simulink model "MultirotorPathFollowing"  (R2025b)
settings: Solver=FixedStepAuto  StartTime=0.0  StopTime=5  FixedStep=1e-4  RelTol=1e-3
undefined symbols (not defined in the file): convertStringsToChars, initialState
libraries: slpidlib x3, uavutilslib x1, uavalgslib x1
settings Model: SimulationMode=accelerator  Creator=Admin  LastModifiedBy=Admin

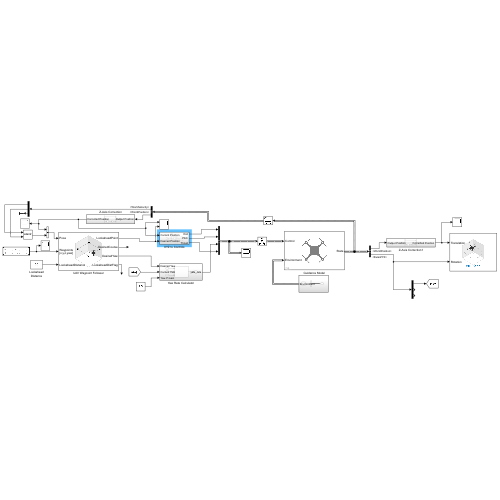
[thumbnail: Simulink's stored preview of the top-level diagram]
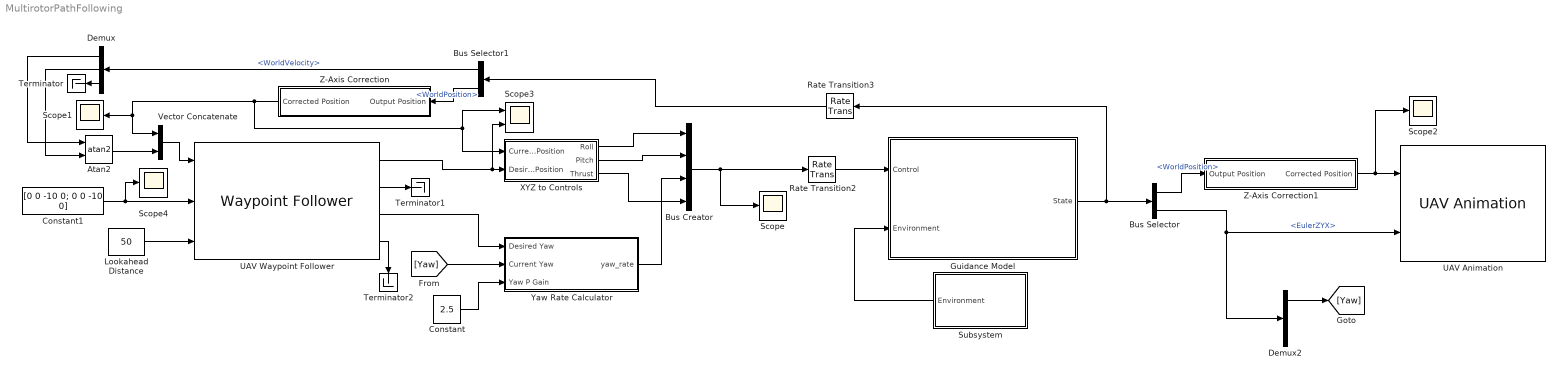
== system MultirotorPathFollowing ==
  Atan2 : Trigonometry  Operator=atan2
  Bus Creator : BusCreator  Inputs=4  OutDataTypeStr=Bus: MultirotorGuidanceControlBus  NonVirtualBus=on
      settings: InheritFromInputs=off
  Bus Selector : BusSelector  OutputSignals=WorldPosition,EulerZYX
  Bus Selector1 : BusSelector  OutputSignals=WorldVelocity,WorldPosition
  Constant : Constant  Value=2.5
  Constant1 : Constant  Value=[0 0 -10 0; 0 0 -10 0]  OutDataTypeStr=Inherit: Inherit via back propagation  SampleTime=-1
  Demux : Demux  Outputs=3
  Demux2 : Demux  Outputs=3
  Guidance Model : Subsystem  AncestorBlock=uavalgslib/Guidance Model  mask(Guidance Model){ModelType=MultirotorGuidance, NumInstances=1, SpecifiedDataType=double, SimulateUsing=Interpreted execution, InitialWorldPositionMultirotor=[0; 0; 10], InitialWorldVelocityMultirotor=[0; 0; 0], InitialEulerZYXMultirotor=[0; 0; 0], InitialBodyAngularRateRPYMultirotor=[0; 0; 0], InitialThrustMultirotor=0, InitialNorthFixedWing=0, InitialEastFixedWing=0, InitialHeightFixedWing=0, InitialAirSpeedFixedWing=0, InitialHeadingAngleFixedWing=0, InitialFlightPathAngleFixedWing=0, InitialRollAngleFixedWing=0, InitialRollAngleRateFixedWing=0, PDRollMultirotor=[3402.97,116.67], PDPitchMultirotor=[3402.97, 116.67], PYawRateMultirotor=1950, PThrustMultirotor=3900, MassMultirotor=2, PHeightFixedWing=3.9, PHeadingAngleFixedWing=3.9, PFlightPathAngleFixedWing=39, PDRollFixedWing=[3402.97, 116.67], PAirSpeedFixedWing=1, FlightPathAngleLimitsFixedWing=[-pi/2, pi/2], StateBusName='MultirotorGuidanceStateBus', ControlBusName='MultirotorGuidanceControlBus', EnvironmentBusName='MultirotorGuidanceEnvironmentBus', DataType=double}
      mask prompts: ModelType "uav:robotsluav:guidancemodelblock:ModelType"; NumInstances "Number of Instances:"; SpecifiedDataType "uav:robotsluav:guidancemodelblock:DataType"; SimulateUsing "SystemBlock:MATLABSystem:SimulateUsing"; InitialWorldPositionMultirotor "uav:robotsluav:guidancemodelblock:WorldPosition"; InitialWorldVelocityMultirotor "uav:robotsluav:guidancemodelblock:WorldVelocity"; InitialEulerZYXMultirotor "uav:robotsluav:guidancemodelblock:EulerZYX"; InitialBodyAngularRateRPYMultirotor "uav:robotsluav:guidancemodelblock:BodyAngularRateRPY"; InitialThrustMultirotor "uav:robotsluav:guidancemodelblock:Thrust"; InitialNorthFixedWing "uav:robotsluav:guidancemodelblock:NorthPosition"; InitialEastFixedWing "uav:robotsluav:guidancemodelblock:EastPosition"; InitialHeightFixedWing "uav:robotsluav:guidancemodelblock:Height"; InitialAirSpeedFixedWing "uav:robotsluav:guidancemodelblock:AirSpeed"; InitialHeadingAngleFixedWing "uav:robotsluav:guidancemodelblock:HeadingAngle"; InitialFlightPathAngleFixedWing "uav:robotsluav:guidancemodelblock:FlightPathAngle"; InitialRollAngleFixedWing "uav:robotsluav:guidancemodelblock:RollAngle"; InitialRollAngleRateFixedWing "uav:robotsluav:guidancemodelblock:RollAngleRate"; PDRollMultirotor "uav:robotsluav:guidancemodelblock:PDRoll"; PDPitchMultirotor "uav:robotsluav:guidancemodelblock:PDPitch"; PYawRateMultirotor "uav:robotsluav:guidancemodelblock:PYawRate"; PThrustMultirotor "uav:robotsluav:guidancemodelblock:PThrust"; MassMultirotor "uav:robotsluav:guidancemodelblock:Mass"; PHeightFixedWing "uav:robotsluav:guidancemodelblock:PHeight"; PHeadingAngleFixedWing "uav:robotsluav:guidancemodelblock:PHeadingAngle"; PFlightPathAngleFixedWing "uav:robotsluav:guidancemodelblock:PFlightPathAngle"; PDRollFixedWing "uav:robotsluav:guidancemodelblock:PDRollAngle"; PAirSpeedFixedWing "uav:robotsluav:guidancemodelblock:PAirSpeed"; FlightPathAngleLimitsFixedWing "uav:robotsluav:guidancemodelblock:MinMaxFlightPathAngle"; StateBusName "uav:robotsluav:guidancemodelblock:StateBusName"; ControlBusName "uav:robotsluav:guidancemodelblock:ControlBusName"; EnvironmentBusName "uav:robotsluav:guidancemodelblock:EnvironmentBusName"; DataType "uav:robotsluav:guidancemodelblock:ResolvedDataType"
      mask help: uav:robotsluav:guidancemodelblock:Description
      mask init:
      | ModelName = gcb;
      | 
      | % Validate bus names
      | uav.sluav.internal.guidancemodel.mask.validateBusNames(gcb);
      | 
      | [stateDimension, initialState, UAVType, UAVDataType, UAVConfig] = ...
      |     uav.sluav.internal.guidancemodel.mask.initialize(ModelName, ModelType, gcb, NumInstances);
      mask Help: eval('helpview(''uav'', ''uavGuidanceModelBlock'')');
      mask TypeOptions ModelType: uav:robotsluav:guidancemodelblock:ModelTypeMultirotor | uav:robotsluav:guidancemodelblock:ModelTypeFixedWing
      mask Callback ModelType:
      | % Change mask dialog
      | uav.sluav.internal.guidancemodel.mask.modelTypeCallback(gcb);
      | 
      | % Create buses for the UAV block
      | uav.sluav.internal.guidancemodel.mask.createUAVBuses(gcb);
      mask Callback SpecifiedDataType:
      | if ~strcmp(get_param(gcb, 'SpecifiedDataType'), '<data type expression>')
      |     % Resolve input type
      |     uav.sluav.internal.guidancemodel.mask.dataTypeCallback(gcb);
      | 
      |     % Create buses for the UAV block
      |     uav.sluav.internal.guidancemodel.mask.createUAVBuses(gcb);
      | end
      mask TypeOptions SimulateUsing: ComputeDerivative/SimulateUsing | StateVector2Struct/SimulateUsing
      mask Callback StateBusName:
      | % Validate bus names
      | uav.sluav.internal.guidancemodel.mask.validateBusNames(gcb);
      | 
      | % Create buses for the UAV block
      | uav.sluav.internal.guidancemodel.mask.createUAVBuses(gcb);
      mask Callback ControlBusName:
      | % Validate bus names
      | uav.sluav.internal.guidancemodel.mask.validateBusNames(gcb);
      | 
      | % Create buses for the UAV block
      | uav.sluav.internal.guidancemodel.mask.createUAVBuses(gcb);
      mask Callback EnvironmentBusName:
      | % Validate bus names
      | uav.sluav.internal.guidancemodel.mask.validateBusNames(gcb);
      | 
      | % Create buses for the UAV block
      | uav.sluav.internal.guidancemodel.mask.createUAVBuses(gcb);
      mask DialogControl ModelType Prompt: Model Type:
      mask DialogControl SpecifiedDataType Prompt: Data Type:
      mask DialogControl SimulateUsing Prompt: Simulate using:
      mask DialogControl SimulateUsing Tooltip: SystemBlock:MATLABSystem:SimulateUsingDescription
      mask DialogControl InitialStateTab Prompt: uav:robotsluav:guidancemodelblock:InitialState
      mask DialogControl InitialWorldPositionMultirotor Prompt: World Position
      mask DialogControl InitialWorldVelocityMultirotor Prompt: World Velocity
      mask DialogControl InitialEulerZYXMultirotor Prompt: Euler Angles (ZYX)
      mask DialogControl InitialBodyAngularRateRPYMultirotor Prompt: Body Angular Rate
      mask DialogControl InitialThrustMultirotor Prompt: Thrust
      mask DialogControl InitialNorthFixedWing Prompt: North Position
      mask DialogControl InitialEastFixedWing Prompt: East Position
      mask DialogControl InitialHeightFixedWing Prompt: Height
      mask DialogControl InitialAirSpeedFixedWing Prompt: Air Speed
      mask DialogControl InitialHeadingAngleFixedWing Prompt: Heading Angle
      mask DialogControl InitialFlightPathAngleFixedWing Prompt: Flight Path Angle
      mask DialogControl InitialRollAngleFixedWing Prompt: Roll Angle
      mask DialogControl InitialRollAngleRateFixedWing Prompt: Roll Angular Velocity
      mask DialogControl ConfigurationTab Prompt: uav:robotsluav:guidancemodelblock:Configuration
      mask DialogControl PDRollMultirotor Prompt: PD Roll
      mask DialogControl PDPitchMultirotor Prompt: PD Pitch
      mask DialogControl PYawRateMultirotor Prompt: P YawRate
      mask DialogControl PThrustMultirotor Prompt: P Thrust
      mask DialogControl MassMultirotor Prompt: Mass
      mask DialogControl PHeightFixedWing Prompt: P Height
      mask DialogControl PHeadingAngleFixedWing Prompt: P Heading Angle
      mask DialogControl PFlightPathAngleFixedWing Prompt: P Flight Path Angle
      mask DialogControl PDRollFixedWing Prompt: PD Roll Angle
      mask DialogControl PAirSpeedFixedWing Prompt: P Air Speed
      mask DialogControl FlightPathAngleLimitsFixedWing Prompt: Min/Max Flight Path Angle
      mask DialogControl BusNameTab Prompt: uav:robotsluav:guidancemodelblock:InputOutputBusNames
      mask DialogControl StateBusName Prompt: State Bus Name
      mask DialogControl ControlBusName Prompt: Control Bus Name
      mask DialogControl EnvironmentBusName Prompt: Environment Bus Name
      mask DialogControl DataType Prompt: Resolved Data Type
      mask Display:
      | port_label('input', 1, 'Control')
      | port_label('input', 2, 'Environment')
      | port_label('output', 1, 'State')
  Lookahead Distance : Constant  Value=50
  Rate Transition2 : RateTransition  OutPortSampleTime=0.1
  Rate Transition3 : RateTransition  OutPortSampleTime=0.1
  Scope{,1..2,4} (4 alike) : Scope
      Scope settings: ActiveDisplayYMinimum=-1  ActiveDisplayYMaximum=1
      Scope1 settings: ActiveDisplayYMinimum=-1  ActiveDisplayYMaximum=1
      Scope2 settings: ActiveDisplayYMinimum=-1  ActiveDisplayYMaximum=1  DataLoggingVariableName=ScopeData2
      Scope4 settings: ActiveDisplayYMinimum=-2.4999999999999996  ActiveDisplayYMaximum=22.5  DataLoggingVariableName=ScopeData4
  Scope3 : Scope  NumInputPorts=2
      settings: ActiveDisplayYMinimum=-481.410610510493  ActiveDisplayYMaximum=53.490067834499207  DataLoggingVariableName=ScopeData3
  Subsystem : Subsystem
  Terminator : Terminator
  Terminator1 : Terminator
  Terminator2 : Terminator
  UAV Animation : uavutilslib/UAV Animation  NumUAV=1  DynamicUAVConfig=off  UAVType=Multirotor  UAVSize=1  UAVColor=[1 0 0]  UAVTrajectoryAlpha=1  InertialZDirection=Down  RotationFormat=Euler ZYX  DrawMarkers=off  SampleTime=-1
  UAV Waypoint Follower : uavalgslib/Waypoint Follower  UAVType=multirotor  StartFrom=first  TransitionRadiusSource=internal  TransitionRadius=10  MinLookaheadDistance=0.1  HoverAtLastWaypoint=off  YawInput=on  ShowCrossTrackErrorOutput=off  ShowStatusOutput=off  SimulateUsing=Code generation
  Vector Concatenate : Concatenate
  XYZ to Controls : Subsystem
  Yaw Rate Calculator : Subsystem
  Z-Axis Correction : Subsystem
  Z-Axis Correction1 : Subsystem
  wires:
  Subsystem/1(Environment) -> Guidance Model/2(Environment)
  Rate Transition2/1 -> Guidance Model/1(Control)
  Guidance Model/1(State) -> Rate Transition3/1, Bus Selector/1
  Bus Selector/2 -> Demux2/1, UAV Animation/2  "<EulerZYX>"
  Lookahead Distance/1 -> UAV Waypoint Follower/3
  Rate Transition3/1 -> Bus Selector1/1
  Vector Concatenate/1 -> UAV Waypoint Follower/1
  Bus Selector1/1 -> Demux/1  "<WorldVelocity>"
  Demux/1 -> Atan2/1
  Demux/2 -> Atan2/2
  Atan2/1 -> Vector Concatenate/2
  Demux/3 -> Terminator/1
  UAV Waypoint Follower/4 -> Terminator2/1
  Bus Creator/1 -> Scope/1, Rate Transition2/1
  UAV Waypoint Follower/3 -> Yaw Rate Calculator/1(Desired Yaw)
  Demux2/1 -> [Yaw]
  [Yaw] -> Yaw Rate Calculator/2("Current Yaw ")
  Constant/1 -> Yaw Rate Calculator/3(Yaw P Gain)
  Yaw Rate Calculator/1(yaw_rate) -> Bus Creator/3
  UAV Waypoint Follower/1 -> Scope3/2, XYZ to Controls/2(Desired Position)
  XYZ to Controls/1(Roll) -> Bus Creator/1
  XYZ to Controls/2(Pitch) -> Bus Creator/2
  XYZ to Controls/3(Thrust) -> Bus Creator/4
  Constant1/1 -> Scope4/1, UAV Waypoint Follower/2
  Bus Selector1/2 -> Z-Axis Correction/1(Output Position)  "<WorldPosition>"
  Z-Axis Correction/1(Corrected Position) -> Scope3/1, XYZ to Controls/1(Current Position), Scope1/1, Vector Concatenate/1
  Z-Axis Correction1/1(Corrected Position) -> Scope2/1, UAV Animation/1
  Bus Selector/1 -> Z-Axis Correction1/1(Output Position)  "<WorldPosition>"
  UAV Waypoint Follower/2 -> Terminator1/1

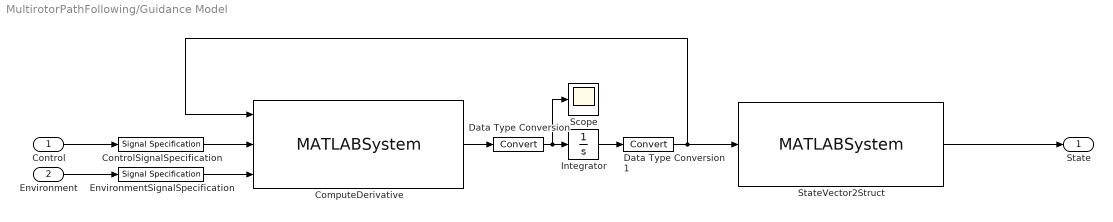
== system MultirotorPathFollowing/Guidance Model ==
  Control : Inport
  Environment : Inport  Port=2
  ComputeDerivative : MATLABSystem  System=robotics.core.internal.system.navigation.Model  ModelName=ModelName  ModelType=UAVType  ModelConfiguration=UAVConfig  DataType=UAVDataType  UseExternalConfiguration=false  NumInstances=NumInstances  SimulateUsing=Interpreted execution
      mask Type: robotics.core.internal.system.navigation.Model
  ControlSignalSpecification : SignalSpecification  OutDataTypeStr=Bus: MultirotorGuidanceControlBus  BusOutputAsStruct=on
  Data Type Conversion : DataTypeConversion  SaturateOnIntegerOverflow=off  RndMeth=Floor
  Data Type Conversion1 : DataTypeConversion  SaturateOnIntegerOverflow=off  RndMeth=Floor
  EnvironmentSignalSpecification : SignalSpecification  OutDataTypeStr=Bus: MultirotorGuidanceEnvironmentBus  BusOutputAsStruct=on
  Integrator : Integrator  InitialCondition=double(initialState)
  Scope : Scope
      settings: ActiveDisplayYMinimum=-20321.068651257519  ActiveDisplayYMaximum=4289.4123209348782  DataLoggingVariableName=ScopeData6
  StateVector2Struct : MATLABSystem  System=robotics.core.internal.system.navigation.StateVector2Struct  OutputBusName=convertStringsToChars(StateBusName)  ModelType=UAVType  DataType=UAVDataType  NumInstances=NumInstances  SimulateUsing=Interpreted execution
      mask Type: robotics.core.internal.system.navigation.StateVector2Struct
  State : Outport  VectorParamsAs1DForOutWhenUnconnected=off  BusOutputAsStruct=on
  wires:
  EnvironmentSignalSpecification/1 -> ComputeDerivative/3
  ControlSignalSpecification/1 -> ComputeDerivative/2
  Data Type Conversion1/1 -> ComputeDerivative/1, StateVector2Struct/1
  Data Type Conversion/1 -> Scope/1, Integrator/1
  Environment/1 -> EnvironmentSignalSpecification/1
  Control/1 -> ControlSignalSpecification/1
  Integrator/1 -> Data Type Conversion1/1
  ComputeDerivative/1 -> Data Type Conversion/1
  StateVector2Struct/1 -> State/1

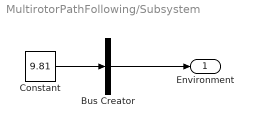
== system MultirotorPathFollowing/Subsystem ==
  Bus Creator : BusCreator  Inputs=1  OutDataTypeStr=Bus: MultirotorGuidanceEnvironmentBus  NonVirtualBus=on
      settings: InheritFromInputs=off
  Constant : Constant  Value=9.81
  Environment : Outport
  wires:
  Bus Creator/1 -> Environment/1
  Constant/1 -> Bus Creator/1

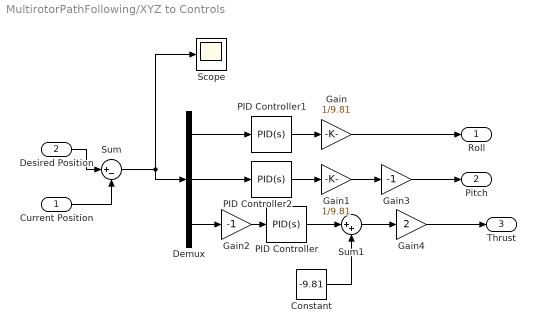
== system MultirotorPathFollowing/XYZ to Controls ==
  Current Position : Inport
  Desired Position : Inport  Port=2
  Constant : Constant  Value=-9.81
  Demux : Demux  Outputs=3
  Gain : Gain  Gain=1/9.81
  Gain1 : Gain  Gain=1/9.81
  Gain2 : Gain  Gain=-1
  Gain3 : Gain  Gain=-1
  Gain4 : Gain  Gain=2
  PID Controller : slpidlib/PID Controller  Controller=PID  Form=Parallel  TimeDomain=Continuous-time  UseExternalTs=off  SampleTime=-1  IntegratorMethod=Forward Euler  FilterMethod=Forward Euler  ControllerParametersSource=internal  P=3  I=0  UseKiTs=off  D=3  UseExternalDerivativeSource=off  N=100  UseFilter=on  TunerSelectOption=Transfer Function Based (PID Tuner App)  InitialConditionSource=internal  InitialConditionForIntegrator=0  InitialConditionForFilter=0  DifferentiatorICPrevScaledInput=0  ExternalReset=none  TrackingMode=off  Kt=1  LimitOutput=off  SatLimitsSource=internal  UpperSaturationLimit=inf  LowerSaturationLimit=-inf  LinearizeAsGain=on  AntiWindupMode=none  Kb=1  LimitIntegrator=off  UpperIntegratorSaturationLimit=inf  LowerIntegratorSaturationLimit=-inf  POutMin=[]  POutMax=[]  IOutMin=[]  IOutMax=[]  DOutMin=[]  DOutMax=[]  NOutMin=[]  NOutMax=[]  SumOutMin=[]  SumOutMax=[]  SaturationOutMin=[]  SaturationOutMax=[]  PParamMin=[]  PParamMax=[]  IParamMin=[]  IParamMax=[]  DParamMin=[]  DParamMax=[]  NParamMin=[]  NParamMax=[]  KbParamMin=[]  KbParamMax=[]  KtParamMin=[]  KtParamMax=[]  KbOutMin=[]  KbOutMax=[]  KtOutMin=[]  KtOutMax=[]  IntegratorOutMin=[]  IntegratorOutMax=[]  FilterOutMin=[]  FilterOutMax=[]  SumI1OutMin=[]  SumI1OutMax=[]  SumI2OutMin=[]  SumI2OutMax=[]  SumI3OutMin=[]  SumI3OutMax=[]  SumI4OutMin=[]  SumI4OutMax=[]  SumDOutMin=[]  SumDOutMax=[]  DifferentiatorOutMin=[]  DifferentiatorOutMax=[]  FilterDiffOutCoefMin=[]  FilterDiffOutCoefMax=[]  ReciprocalOutMin=[]  ReciprocalOutMax=[]  SumDenOutMin=[]  SumDenOutMax=[]  SumNumOutMin=[]  SumNumOutMax=[]  DivideOutMin=[]  DivideOutMax=[]  UdiffTsProdOutMin=[]  UdiffTsProdOutMax=[]  NTsProdOutMin=[]  NTsProdOutMax=[]  UintegralTsProdOutMin=[]  UintegralTsProdOutMax=[]  UngainTsProdOutMin=[]  UngainTsProdOutMax=[]  ClampingZeroOutDataTypeStr=Inherit: Inherit via back propagation  ClampingZeroOutMin=[]  ClampingZeroOutMax=[]  FilterDenConstantOutDataTypeStr=Inherit: Inherit via back propagation  FilterDenConstantOutMin=[]  FilterDenConstantOutMax=[]  PCopyOutDataTypeStr=Inherit: Inherit via back propagation  PCopyOutMin=[]  PCopyOutMax=[]  NCopyOutDataTypeStr=Inherit: Inherit via back propagation  NCopyOutMin=[]  NCopyOutMax=[]  IntegratorContinuousStateAttributes=''  IntegratorStateMustResolveToSignalObject=off  IntegratorRTWStateStorageClass=Auto  FilterContinuousStateAttributes=''  FilterStateMustResolveToSignalObject=off  FilterRTWStateStorageClass=Auto  ParallelPVariant=InternalParameters  IdealPVariant=Disabled  IVariant=InternalParameters  DVariant=InternalParameters  IntegratorVariant=Continuous  SatVariant=Disabled  AWVariant=Passthrough  PCopyVariant=Disabled  TRVariant=Disabled  FdbkBlocksVariant=Forward  IdealPFdbkVariant=Disabled  SatFdbkVariant=Disabled  DerivativeFilterVariant=ContFilter  NVariant=InternalParameters  NCopyVariant=Disabled  FilterICVariant=InternalICsFilter  IntegratorICVariant=InternalICs  ExternalResetVariant=Disabled  TRSumVariant=Passthrough  SumFdbkVariant=Disabled  SumVariant=Sum_PID  TsampFilterVariant=InternalTs  TsampNgainVariant=Passthrough  TsampIntegralVariant=Disabled_SignalSpec  ExternalSaturationOutDataTypeStr=Inherit: Same as second input  DerivativeSourceVariant=ErrorSignal  PreIntVariant=InternalPreInt
  PID Controller1 : slpidlib/PID Controller  Controller=PID  Form=Parallel  TimeDomain=Continuous-time  UseExternalTs=off  SampleTime=-1  IntegratorMethod=Forward Euler  FilterMethod=Forward Euler  ControllerParametersSource=internal  P=1  I=0  UseKiTs=off  D=1  UseExternalDerivativeSource=off  N=100  UseFilter=on  TunerSelectOption=Transfer Function Based (PID Tuner App)  InitialConditionSource=internal  InitialConditionForIntegrator=0  InitialConditionForFilter=0  DifferentiatorICPrevScaledInput=0  ExternalReset=none  TrackingMode=off  Kt=1  LimitOutput=off  SatLimitsSource=internal  UpperSaturationLimit=inf  LowerSaturationLimit=-inf  LinearizeAsGain=on  AntiWindupMode=none  Kb=1  LimitIntegrator=off  UpperIntegratorSaturationLimit=inf  LowerIntegratorSaturationLimit=-inf  POutMin=[]  POutMax=[]  IOutMin=[]  IOutMax=[]  DOutMin=[]  DOutMax=[]  NOutMin=[]  NOutMax=[]  SumOutMin=[]  SumOutMax=[]  SaturationOutMin=[]  SaturationOutMax=[]  PParamMin=[]  PParamMax=[]  IParamMin=[]  IParamMax=[]  DParamMin=[]  DParamMax=[]  NParamMin=[]  NParamMax=[]  KbParamMin=[]  KbParamMax=[]  KtParamMin=[]  KtParamMax=[]  KbOutMin=[]  KbOutMax=[]  KtOutMin=[]  KtOutMax=[]  IntegratorOutMin=[]  IntegratorOutMax=[]  FilterOutMin=[]  FilterOutMax=[]  SumI1OutMin=[]  SumI1OutMax=[]  SumI2OutMin=[]  SumI2OutMax=[]  SumI3OutMin=[]  SumI3OutMax=[]  SumI4OutMin=[]  SumI4OutMax=[]  SumDOutMin=[]  SumDOutMax=[]  DifferentiatorOutMin=[]  DifferentiatorOutMax=[]  FilterDiffOutCoefMin=[]  FilterDiffOutCoefMax=[]  ReciprocalOutMin=[]  ReciprocalOutMax=[]  SumDenOutMin=[]  SumDenOutMax=[]  SumNumOutMin=[]  SumNumOutMax=[]  DivideOutMin=[]  DivideOutMax=[]  UdiffTsProdOutMin=[]  UdiffTsProdOutMax=[]  NTsProdOutMin=[]  NTsProdOutMax=[]  UintegralTsProdOutMin=[]  UintegralTsProdOutMax=[]  UngainTsProdOutMin=[]  UngainTsProdOutMax=[]  ClampingZeroOutDataTypeStr=Inherit: Inherit via back propagation  ClampingZeroOutMin=[]  ClampingZeroOutMax=[]  FilterDenConstantOutDataTypeStr=Inherit: Inherit via back propagation  FilterDenConstantOutMin=[]  FilterDenConstantOutMax=[]  PCopyOutDataTypeStr=Inherit: Inherit via back propagation  PCopyOutMin=[]  PCopyOutMax=[]  NCopyOutDataTypeStr=Inherit: Inherit via back propagation  NCopyOutMin=[]  NCopyOutMax=[]  IntegratorContinuousStateAttributes=''  IntegratorStateMustResolveToSignalObject=off  IntegratorRTWStateStorageClass=Auto  FilterContinuousStateAttributes=''  FilterStateMustResolveToSignalObject=off  FilterRTWStateStorageClass=Auto  ParallelPVariant=InternalParameters  IdealPVariant=Disabled  IVariant=InternalParameters  DVariant=InternalParameters  IntegratorVariant=Continuous  SatVariant=Disabled  AWVariant=Passthrough  PCopyVariant=Disabled  TRVariant=Disabled  FdbkBlocksVariant=Forward  IdealPFdbkVariant=Disabled  SatFdbkVariant=Disabled  DerivativeFilterVariant=ContFilter  NVariant=InternalParameters  NCopyVariant=Disabled  FilterICVariant=InternalICsFilter  IntegratorICVariant=InternalICs  ExternalResetVariant=Disabled  TRSumVariant=Passthrough  SumFdbkVariant=Disabled  SumVariant=Sum_PID  TsampFilterVariant=InternalTs  TsampNgainVariant=Passthrough  TsampIntegralVariant=Disabled_SignalSpec  ExternalSaturationOutDataTypeStr=Inherit: Same as second input  DerivativeSourceVariant=ErrorSignal  PreIntVariant=InternalPreInt
  PID Controller2 : slpidlib/PID Controller  Controller=PID  Form=Parallel  TimeDomain=Continuous-time  UseExternalTs=off  SampleTime=-1  IntegratorMethod=Forward Euler  FilterMethod=Forward Euler  ControllerParametersSource=internal  P=1  I=0  UseKiTs=off  D=1  UseExternalDerivativeSource=off  N=100  UseFilter=on  TunerSelectOption=Transfer Function Based (PID Tuner App)  InitialConditionSource=internal  InitialConditionForIntegrator=0  InitialConditionForFilter=0  DifferentiatorICPrevScaledInput=0  ExternalReset=none  TrackingMode=off  Kt=1  LimitOutput=off  SatLimitsSource=internal  UpperSaturationLimit=inf  LowerSaturationLimit=-inf  LinearizeAsGain=on  AntiWindupMode=none  Kb=1  LimitIntegrator=off  UpperIntegratorSaturationLimit=inf  LowerIntegratorSaturationLimit=-inf  POutMin=[]  POutMax=[]  IOutMin=[]  IOutMax=[]  DOutMin=[]  DOutMax=[]  NOutMin=[]  NOutMax=[]  SumOutMin=[]  SumOutMax=[]  SaturationOutMin=[]  SaturationOutMax=[]  PParamMin=[]  PParamMax=[]  IParamMin=[]  IParamMax=[]  DParamMin=[]  DParamMax=[]  NParamMin=[]  NParamMax=[]  KbParamMin=[]  KbParamMax=[]  KtParamMin=[]  KtParamMax=[]  KbOutMin=[]  KbOutMax=[]  KtOutMin=[]  KtOutMax=[]  IntegratorOutMin=[]  IntegratorOutMax=[]  FilterOutMin=[]  FilterOutMax=[]  SumI1OutMin=[]  SumI1OutMax=[]  SumI2OutMin=[]  SumI2OutMax=[]  SumI3OutMin=[]  SumI3OutMax=[]  SumI4OutMin=[]  SumI4OutMax=[]  SumDOutMin=[]  SumDOutMax=[]  DifferentiatorOutMin=[]  DifferentiatorOutMax=[]  FilterDiffOutCoefMin=[]  FilterDiffOutCoefMax=[]  ReciprocalOutMin=[]  ReciprocalOutMax=[]  SumDenOutMin=[]  SumDenOutMax=[]  SumNumOutMin=[]  SumNumOutMax=[]  DivideOutMin=[]  DivideOutMax=[]  UdiffTsProdOutMin=[]  UdiffTsProdOutMax=[]  NTsProdOutMin=[]  NTsProdOutMax=[]  UintegralTsProdOutMin=[]  UintegralTsProdOutMax=[]  UngainTsProdOutMin=[]  UngainTsProdOutMax=[]  ClampingZeroOutDataTypeStr=Inherit: Inherit via back propagation  ClampingZeroOutMin=[]  ClampingZeroOutMax=[]  FilterDenConstantOutDataTypeStr=Inherit: Inherit via back propagation  FilterDenConstantOutMin=[]  FilterDenConstantOutMax=[]  PCopyOutDataTypeStr=Inherit: Inherit via back propagation  PCopyOutMin=[]  PCopyOutMax=[]  NCopyOutDataTypeStr=Inherit: Inherit via back propagation  NCopyOutMin=[]  NCopyOutMax=[]  IntegratorContinuousStateAttributes=''  IntegratorStateMustResolveToSignalObject=off  IntegratorRTWStateStorageClass=Auto  FilterContinuousStateAttributes=''  FilterStateMustResolveToSignalObject=off  FilterRTWStateStorageClass=Auto  ParallelPVariant=InternalParameters  IdealPVariant=Disabled  IVariant=InternalParameters  DVariant=InternalParameters  IntegratorVariant=Continuous  SatVariant=Disabled  AWVariant=Passthrough  PCopyVariant=Disabled  TRVariant=Disabled  FdbkBlocksVariant=Forward  IdealPFdbkVariant=Disabled  SatFdbkVariant=Disabled  DerivativeFilterVariant=ContFilter  NVariant=InternalParameters  NCopyVariant=Disabled  FilterICVariant=InternalICsFilter  IntegratorICVariant=InternalICs  ExternalResetVariant=Disabled  TRSumVariant=Passthrough  SumFdbkVariant=Disabled  SumVariant=Sum_PID  TsampFilterVariant=InternalTs  TsampNgainVariant=Passthrough  TsampIntegralVariant=Disabled_SignalSpec  ExternalSaturationOutDataTypeStr=Inherit: Same as second input  DerivativeSourceVariant=ErrorSignal  PreIntVariant=InternalPreInt
  Scope : Scope
      settings: ActiveDisplayYMinimum=-56.250000000000028  ActiveDisplayYMaximum=6.2500000000000018  DataLoggingVariableName=ScopeData5
  Sum : Sum  Inputs=|+-
  Sum1 : Sum  Inputs=|++
  Roll : Outport
  Pitch : Outport  Port=2
  Thrust : Outport  Port=3
  wires:
  Desired Position/1 -> Sum/1
  Current Position/1 -> Sum/2
  Sum/1 -> Demux/1, Scope/1
  Demux/3 -> Gain2/1
  Gain2/1 -> PID Controller/1
  Demux/1 -> PID Controller1/1
  PID Controller1/1 -> Gain/1
  Gain/1 -> Roll/1
  PID Controller2/1 -> Gain1/1
  Demux/2 -> PID Controller2/1
  Gain1/1 -> Gain3/1
  Gain3/1 -> Pitch/1
  Constant/1 -> Sum1/2
  PID Controller/1 -> Sum1/1
  Sum1/1 -> Gain4/1
  Gain4/1 -> Thrust/1

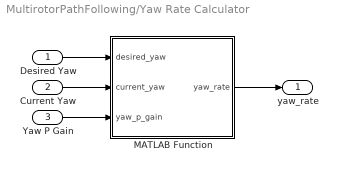
== system MultirotorPathFollowing/Yaw Rate Calculator ==
  Desired Yaw : Inport
  "Current Yaw " : Inport  Port=2
  Yaw P Gain : Inport  Port=3
  MATLAB Function : MATLAB Function  TreatAsAtomicUnit=on
  yaw_rate : Outport
  wires:
  MATLAB Function/1(yaw_rate) -> yaw_rate/1
  Desired Yaw/1 -> MATLAB Function/1(desired_yaw)
  "Current Yaw "/1 -> MATLAB Function/2(current_yaw)
  Yaw P Gain/1 -> MATLAB Function/3(yaw_p_gain)

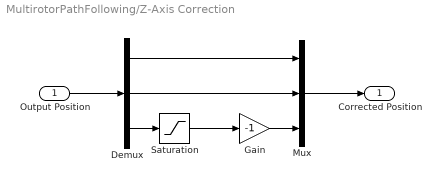
== system MultirotorPathFollowing/Z-Axis Correction ==
  Output Position : Inport
  Demux : Demux  Outputs=3
  Gain : Gain  Gain=-1
  Mux : Mux  Inputs=3
  Saturation : Saturate  UpperLimit=inf  LowerLimit=0
  Corrected Position : Outport
  wires:
  Mux/1 -> Corrected Position/1
  Output Position/1 -> Demux/1
  Demux/1 -> Mux/1
  Demux/2 -> Mux/2
  Gain/1 -> Mux/3
  Demux/3 -> Saturation/1
  Saturation/1 -> Gain/1

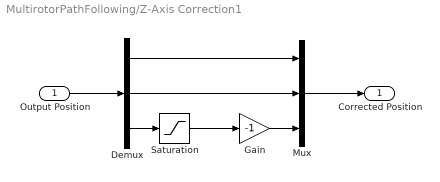
== system MultirotorPathFollowing/Z-Axis Correction1 ==
  Output Position : Inport
  Demux : Demux  Outputs=3
  Gain : Gain  Gain=-1
  Mux : Mux  Inputs=3
  Saturation : Saturate  UpperLimit=inf  LowerLimit=0
  Corrected Position : Outport
  wires:
  Mux/1 -> Corrected Position/1
  Output Position/1 -> Demux/1
  Demux/1 -> Mux/1
  Demux/2 -> Mux/2
  Gain/1 -> Mux/3
  Demux/3 -> Saturation/1
  Saturation/1 -> Gain/1

== matlab function MultirotorPathFollowing/Yaw Rate Calculator/MATLAB Function ==
  data: desired_yaw input; yaw_rate output; current_yaw input; yaw_p_gain input
function yaw_rate = fcn(desired_yaw, current_yaw, yaw_p_gain)

yaw_rate = yaw_p_gain * wrapToPi(desired_yaw - current_yaw);
